simulink model "Palab3_3_6"  (R2025a)
settings: Solver=VariableStepAuto  StartTime=0.0  StopTime=10.0  RelTol=1e-3
settings Model: LastModifiedBy=mieszko

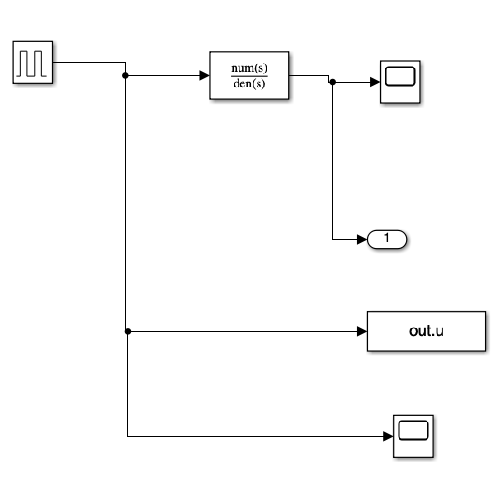
[thumbnail: Simulink's stored preview of the top-level diagram]
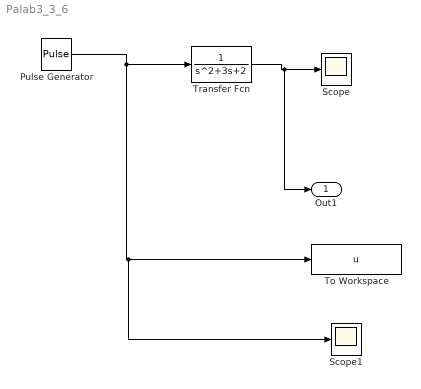
== system Palab3_3_6 ==
  Pulse Generator : DiscretePulseGenerator  PulseType=Time based  Period=6.28  PulseWidth=50
  Scope : Scope
      settings: ActiveDisplayYMinimum=-0.05743  ActiveDisplayYMaximum=0.51688
  Scope1 : Scope
      settings: ActiveDisplayYMinimum=-0.125  ActiveDisplayYMaximum=1.125
  To Workspace : ToWorkspace  VariableName=u  SampleTime=-1
  Transfer Fcn : TransferFcn  Denominator=[1 3 2]
  Out1 : Outport
  wires:
  Pulse Generator/1 -> Scope1/1, To Workspace/1, Transfer Fcn/1
  Transfer Fcn/1 -> Out1/1, Scope/1
